simulink model "aflevering3_simulink"  (R2021b)
settings: Solver=VariableStepAuto  StartTime=0.0  StopTime=1.5  RelTol=1e-3
values from neighbouring files (symbols this model uses):
  A = [0    1.0000         0         0 ... (first row only)    [Controlability.m]    (also in Observability.m = [   0   1   0   0; matlabFile.m = [0  1   0   0;0 -b1/J  0  -b2/J; 0 0 0 1; 0 0 0 -b3/m]; modelleringD.m = a)
  B = [    0 ... (first row only)    [Controlability.m]    (also in Observability.m = [   0; matlabFile.m = [0 0; -r/J r/J; 0 0; 1/m 1/m]; modelleringD.m = b)
  C = [B A*B A^2*B A^3*B]    [Controlability.m]    (also in Observability.m = [ 1   0   0   0; matlabFile.m = [1 0 0 0; 0 0 1 0]; modelleringD.m = c)
  F = Fc*Tinv    [Controlability.m]    (also in matlabFile.m = K(:, 1:4))
  Fi = K(:, [5, 6])    [matlabFile.m]
  L = place(A, B, [-5, -10, -15, -20])    [Observability.m]    (also in matlabFile.m = L')
settings Model: Creator=Simon  LastModifiedBy=fryde
settings SolverCC: AlgebraicLoopSolver=TrustRegion
settings DebuggingCC: SFMachineParentedDataDiag=warning

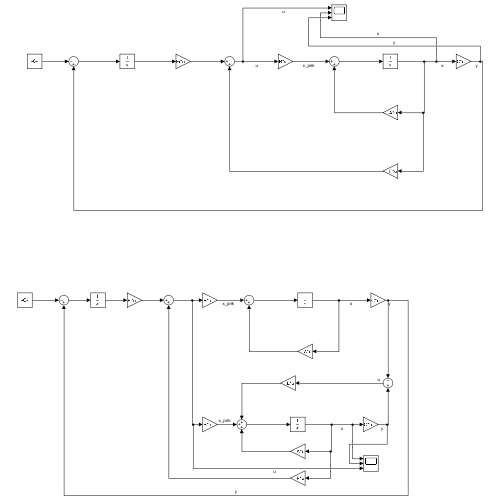
[thumbnail: Simulink's stored preview of the top-level diagram]
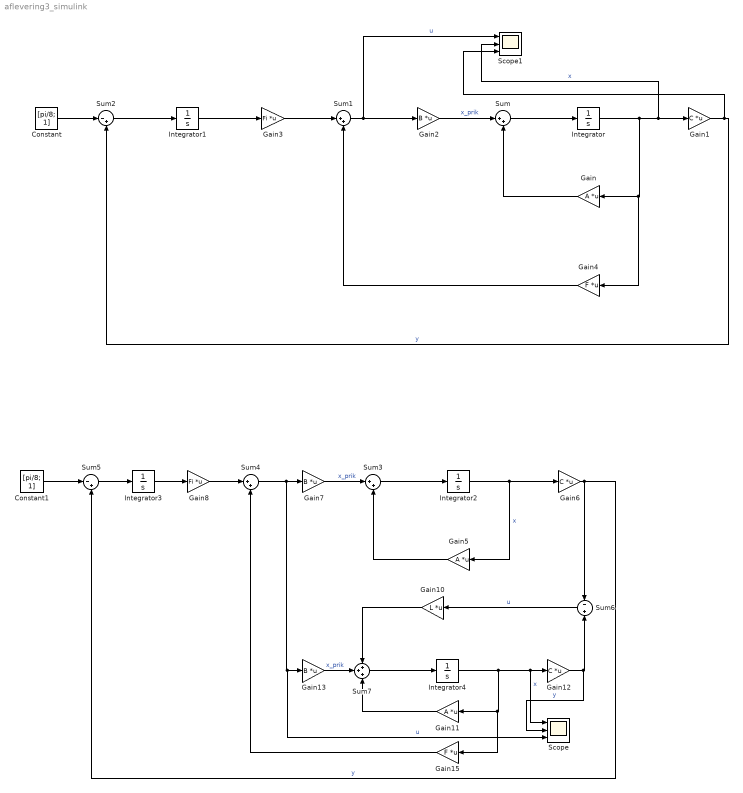
== system aflevering3_simulink ==
  Constant : Constant  Value=[pi/8; 1]  VectorParams1D=off
  Constant1 : Constant  Value=[pi/8; 1]  VectorParams1D=off  SampleTime=0.0001
  Gain : Gain  Gain=A  Multiplication=Matrix(K*u)
  Gain1 : Gain  Gain=C  Multiplication=Matrix(K*u)
  Gain10 : Gain  Gain=L  Multiplication=Matrix(K*u)
  Gain11 : Gain  Gain=A  Multiplication=Matrix(K*u)
  Gain12 : Gain  Gain=C  Multiplication=Matrix(K*u)
  Gain13 : Gain  Gain=B  Multiplication=Matrix(K*u)
  Gain15 : Gain  Gain=F  Multiplication=Matrix(K*u)
  Gain2 : Gain  Gain=B  Multiplication=Matrix(K*u)
  Gain3 : Gain  Gain=Fi  Multiplication=Matrix(K*u)
  Gain4 : Gain  Gain=F  Multiplication=Matrix(K*u)
  Gain5 : Gain  Gain=A  Multiplication=Matrix(K*u)
  Gain6 : Gain  Gain=C  Multiplication=Matrix(K*u)
  Gain7 : Gain  Gain=B  Multiplication=Matrix(K*u)
  Gain8 : Gain  Gain=Fi  Multiplication=Matrix(K*u)
  Integrator{,1..4} (5 alike) : Integrator
  Scope : Scope  NumInputPorts=3
  Scope1 : Scope  NumInputPorts=3
  Sum{,1,3..4} (4 alike) : Sum  Inputs=|++
  Sum2 : Sum  Inputs=|-+
  Sum5 : Sum  Inputs=|-+
  Sum6 : Sum  Inputs=-|+
  Sum7 : Sum  Inputs=+++
  wires:
  Sum/1 -> Integrator/1
  Integrator/1 -> Scope1/2, Gain1/1, Gain4/1, Gain/1  "x"
  Gain2/1 -> Sum/1  "x_prik"
  Sum1/1 -> Scope1/1, Gain2/1  "u"
  Gain/1 -> Sum/2
  Gain3/1 -> Sum1/1
  Integrator1/1 -> Gain3/1
  Sum2/1 -> Integrator1/1
  Gain1/1 -> Scope1/3, Sum2/2  "y"
  Gain4/1 -> Sum1/2
  Constant/1 -> Sum2/1
  Constant1/1 -> Sum5/1
  Gain7/1 -> Sum3/1  "x_prik"
  Integrator2/1 -> Gain6/1, Gain5/1  "x"
  Sum5/1 -> Integrator3/1
  Integrator3/1 -> Gain8/1
  Gain5/1 -> Sum3/2
  Sum3/1 -> Integrator2/1
  Gain6/1 -> Sum6/1, Sum5/2  "y"
  Sum6/1 -> Gain10/1  "u"
  Integrator4/1 -> Scope/1, Gain12/1, Gain15/1, Gain11/1  "x"
  Sum7/1 -> Integrator4/1
  Gain13/1 -> Sum7/2  "x_prik"
  Gain11/1 -> Sum7/3
  Gain10/1 -> Sum7/1
  Gain12/1 -> Scope/2, Sum6/2  "y"
  Gain8/1 -> Sum4/1
  Sum4/1 -> Scope/3, Gain13/1, Gain7/1  "u"
  Gain15/1 -> Sum4/2
